simulink model "BatteryStoragePVPlantGFM"  (R2023a)
settings: Solver=FixedStepDiscrete  StartTime=0.0  StopTime=SimulationTime  RelTol=1e-3
PreLoadFcn:
  | run('BatteryStoragePVPlantGFMParameters')
undefined symbols (not defined in the file): Array, Base, battery, BatteryInverter, DiscIntNeverNeededParam, ee, Feeder, fRT, GFLBatteryController, GFMBatteryController, Grid, GridTransformer, Line, Load, Load2CB_final, Load2CB_initial, LVRT, maxSoC, maxVdc, minIrrad, minSoC, minVdc, Mpp, olTime, Panel, PVController, PVInverter, PVTransformer, Scenario, SM, SubTransmissionLine, Ts, VSMbase
libraries: ee_lib x51, nesl_utility x45, fl_lib x26, eeGeneralControl x18, simulink x12, eeTransforms x11, slpidlib x8, eePowerMeasurement x5, batteryecm_lib x2, eeTotalHarmonicDistorsion x2, spsLeadLagFilterLib x1, eeSmAC1C x1
(part 1 of 5)
Description:
  | Copyright 2022 - 2023 The MathWorks, Inc.
settings Model: SimulationMode=accelerator  Creator=rajarshd  LastModifiedBy=rajarshd
settings DataIOCC: InitialState=op  SaveOutput=off  SaveTime=off  ReturnWorkspaceOutputs=off  SignalLoggingName=logs_ee_spv_park_battery
settings OptimizationCC: ReuseModelBlockBuffer=off
settings ModelReferenceCC: EnableRefExpFcnMdlSchedulingChecks=on
settings SimscapeCC: SimscapeLogType=all  SimscapeLogSimulationStatistics=on  SimscapeLogName=simlog_ee_spv_park_battery  SimscapeLogLimitData=off  SimscapeOperatingPoint=op

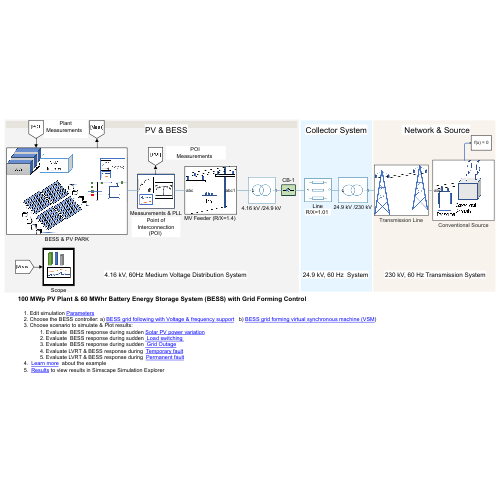
[thumbnail: Simulink's stored preview of the top-level diagram]
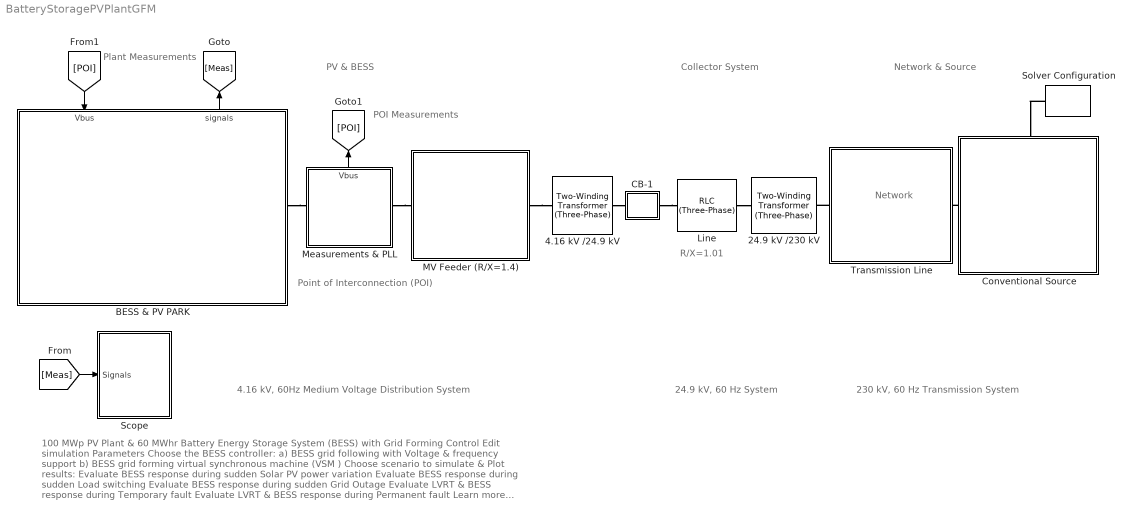
== system BatteryStoragePVPlantGFM ==
  note: Collector System
  note: PV & BESS
  note: Network & Source
  note: Network
  note: 100 MWp PV Plant & 60 MWhr Battery Energy Storage System (BESS) with Grid Forming Control
      |
      | Edit simulation Parameters
      | Choose the BESS controller: a) BESS grid following with Voltage & frequency support b) BESS grid forming virtual synchronous machine (VSM )
      | Choose scenario to simulate & Plot results:
      | Evaluate BESS response during sudden Solar PV power variation
      | Evaluate BESS response during sudden Load switching
      | Evaluate BESS response during sudden Grid Outage
      | Evaluate LVRT & BESS response during Temporary fault
      | Evaluate LVRT & BESS response during Permanent fault
      | Learn more about the example
      | Results to view results in Simscape Simulation Explorer
  note: Point of Interconnection (POI)
  note: 230 kV, 60 Hz Transmission System
  note: 4.16 kV, 60Hz Medium Voltage Distribution System
  note: 24.9 kV, 60 Hz System
  note: R/X=1.01
  note: Plant
      | Measurements
  note: POI
      | Measurements
  24.9 kV /230 kV : ee_lib/Passive/Transformers/Two-Winding Transformer (Three-Phase)  SRated=GridTransformer.VA A*V  FRated=Grid.frequency Hz  Winding1Connection=ee.enum.windingconnection.delta1  VRated1=GridTransformer.hv V  Winding2Connection=ee.enum.windingconnection.Yg  VRated2=GridTransformer.lv V  CoreType=ee.enum.coretype.threelimb  pu_Rw1=GridTransformer.winding_resistance/2  pu_Rw2=GridTransformer.winding_resistance/2  leakage_reactance_option=ee.enum.transformer_leakage.include  pu_Xl1=GridTransformer.winding_lekage_reactance/2  pu_Xl2=GridTransformer.winding_lekage_reactance/2  magnetizing_resistance_option=ee.enum.transformer_magnetizingResistance.exclude  pu_Rm=500  magnetizing_reactance_option=ee.enum.transformer_magnetizingReactance.exclude  saturation_option=ee.enum.transformer_saturation.exclude  pu_Xm=500  current_data=[0, .002, 1, 2]  magnetic_flux_data=[0, 1.2, 1.5, 1.51]  pu_X0=GridTransformer.zero_sequence_reactance  i1_specify=off  i1_priority=None  i1=[0, 0, 0] A  i1_nominal_specify=off  i1_nominal_unit=A  i1_nominal_value=1  i2_specify=off  i2_priority=None  i2=[0, 0, 0] A  i2_nominal_specify=off  i2_nominal_unit=A  i2_nominal_value=1  phi_specify=off  phi_priority=None  phi=[0, 0, 0]  phi_nominal_specify=off  phi_nominal_unit=1  phi_nominal_value=1  power_dissipated_specify=off  power_dissipated_priority=None  power_dissipated=0 W  power_dissipated_nominal_specify=off  power_dissipated_nominal_unit=W  power_dissipated_nominal_value=1
      settings: InternalSimscapePortConfiguration="{\"Bottom\":[],\"Left\":[{\"id\":\"N1\",\"label\":\"~1\",\"type\":\"foundation.electrical.three_phase\"}],\"Right\":[{\"id\":\"N2\",\"label\":\"~2\",\"type\":\"foundation.electrical.three_phase\"}],\"Top\":[]}"
  4.16 kV /24.9 kV : ee_lib/Passive/Transformers/Two-Winding Transformer (Three-Phase)  SRated=PVTransformer.VA A*V  FRated=Grid.frequency Hz  Winding1Connection=ee.enum.windingconnection.delta1  VRated1=PVTransformer.hv V  Winding2Connection=ee.enum.windingconnection.Yg  VRated2=PVTransformer.lv V  CoreType=ee.enum.coretype.threelimb  pu_Rw1=PVTransformer.winding_resistance/2  pu_Rw2=PVTransformer.winding_resistance/2  leakage_reactance_option=ee.enum.transformer_leakage.include  pu_Xl1=PVTransformer.winding_lekage_reactance/2  pu_Xl2=PVTransformer.winding_lekage_reactance/2  magnetizing_resistance_option=ee.enum.transformer_magnetizingResistance.exclude  pu_Rm=500  magnetizing_reactance_option=ee.enum.transformer_magnetizingReactance.exclude  saturation_option=ee.enum.transformer_saturation.exclude  pu_Xm=500  current_data=[0, .002, 1, 2]  magnetic_flux_data=[0, 1.2, 1.5, 1.51]  pu_X0=PVTransformer.zero_sequence_reactance  i1_specify=off  i1_priority=None  i1=[0, 0, 0] A  i1_nominal_specify=off  i1_nominal_unit=A  i1_nominal_value=1  i2_specify=off  i2_priority=None  i2=[0, 0, 0] A  i2_nominal_specify=off  i2_nominal_unit=A  i2_nominal_value=1  phi_specify=off  phi_priority=None  phi=[0, 0, 0]  phi_nominal_specify=off  phi_nominal_unit=1  phi_nominal_value=1  power_dissipated_specify=off  power_dissipated_priority=None  power_dissipated=0 W  power_dissipated_nominal_specify=off  power_dissipated_nominal_unit=W  power_dissipated_nominal_value=1
      settings: InternalSimscapePortConfiguration="{\"Bottom\":[],\"Left\":[{\"id\":\"N1\",\"label\":\"~1\",\"type\":\"foundation.electrical.three_phase\"}],\"Right\":[{\"id\":\"N2\",\"label\":\"~2\",\"type\":\"foundation.electrical.three_phase\"}],\"Top\":[]}"
  BESS & PV PARK : Subsystem
      settings: PortSchema="{\"entries\":[{\"content\":{\"sides\":[{\"content\":{\"connectorIds\":[]},\"type\":\"ConnectorPlacement.EquallySpacedRectSide\",\"uuid\":\"19e6e0fd-37ae-4388-8e0e-5a20feba0fd4\"},{\"content\":{\"connectorIds\":[\"RConn1\"],\"side\":\"RIGHT\"},\"type\":\"ConnectorPlacement.EquallySpacedRectSide\",\"uuid\":\"5a7c928c-05b2-4ad3-8813-df6fbac671b7\"},{\"content\":{\"connectorIds\":[\"In1\",\"Out1\"],\"side\":\"TOP\"},\"type\":\"ConnectorPlacement.EquallySpacedRectSide\",\"uuid\":\"fc17c31c-808c-4646-acd6-16363c98e490\"}]},\"type\":\"ConnectorPlacement.EquallySpacedConnector\",\"uuid\":\"d03db955-298f-40d1-b8c3-c83724e206fe\"}],\"packageUris\":[\"http://schema.mathworks.com/mf0/Connector/R2020b\"],\"version\":\"1.0\"}"
      mask Display: image('$imagefile'); % Use "Edit Image" on toolstrip to change.
  CB-1 : Subsystem
      mask Display: image('$imagefile'); % Use "Edit Image" on toolstrip to change.
  Conventional Source : Subsystem
      settings: PortSchema="{\"entries\":[{\"content\":{\"sides\":[{\"content\":{\"connectorIds\":[\"LConn1\"]},\"type\":\"ConnectorPlacement.EquallySpacedRectSide\",\"uuid\":\"88e24179-6079-4110-b6c8-07285d357c8a\"},{\"content\":{\"connectorIds\":[],\"side\":\"RIGHT\"},\"type\":\"ConnectorPlacement.EquallySpacedRectSide\",\"uuid\":\"8f4b6582-111e-4598-90a5-fa5f81c444ee\"},{\"content\":{\"connectorIds\":[\"LConn2\"],\"side\":\"TOP\"},\"type\":\"ConnectorPlacement.EquallySpacedRectSide\",\"uuid\":\"53212e71-0f3c-4549-bc92-047e88eae9b6\"},{\"content\":{\"connectorIds\":[],\"side\":\"BOTTOM\"},\"type\":\"ConnectorPlacement.EquallySpacedRectSide\",\"uuid\":\"0193069a-d0a5-4b89-8f2a-3f6fb986b7f7\"}]},\"type\":\"ConnectorPlacement.EquallySpacedConnector\",\"uuid\":\"b2543555-7807-483c-9e73-a2cd2a98a3a5\"}],\"packageUris\":[\"http://schema.mathworks.com/mf0/Connector/R2020b\"],\"version\":\"1.0\"}"
      mask Display: image('$imagefile'); % Use "Edit Image" on toolstrip to change.
  Line : ee_lib/Passive/RLC Assemblies/RLC (Three-Phase)  component_structure=ee.enum.rlc.structure.SeriesRL  R=SubTransmissionLine.R*SubTransmissionLine.length Ohm  L=SubTransmissionLine.L*SubTransmissionLine.length H  C=1e-6 F  R_parasitic=0 Ohm  G_parasitic=0 1/Ohm  IL_specify=off  IL_priority=High  IL=[0, 0, 0] A  IL_nominal_specify=off  IL_nominal_unit=A  IL_nominal_value=1  VC_specify=off  VC_priority=High  VC=[0, 0, 0] V  VC_nominal_specify=off  VC_nominal_unit=V  VC_nominal_value=1
      settings: InternalSimscapePortConfiguration="{\"Bottom\":[],\"Left\":[{\"id\":\"N1\",\"label\":\"~1\",\"type\":\"foundation.electrical.three_phase\"}],\"Right\":[{\"id\":\"N2\",\"label\":\"~2\",\"type\":\"foundation.electrical.three_phase\"}],\"Top\":[]}"
  "MV Feeder (R/X=1.4) " : Subsystem
      mask Display: image('$imagefile'); % Use "Edit Image" on toolstrip to change.
  Measurements & PLL : Subsystem
      settings: PortSchema="{\"entries\":[{\"content\":{\"sides\":[{\"content\":{\"connectorIds\":[\"LConn1\"]},\"type\":\"ConnectorPlacement.EquallySpacedRectSide\",\"uuid\":\"0a665b18-901e-42b1-b0d0-6060e0da8e79\"},{\"content\":{\"connectorIds\":[\"RConn1\"],\"side\":\"RIGHT\"},\"type\":\"ConnectorPlacement.EquallySpacedRectSide\",\"uuid\":\"7ff1075b-9d20-42a5-b79b-99217310976a\"},{\"content\":{\"connectorIds\":[\"Out1\"],\"side\":\"TOP\"},\"type\":\"ConnectorPlacement.EquallySpacedRectSide\",\"uuid\":\"7168f638-c3c0-42b4-ab34-d46b363fbd60\"},{\"content\":{\"connectorIds\":[],\"side\":\"BOTTOM\"},\"type\":\"ConnectorPlacement.EquallySpacedRectSide\",\"uuid\":\"9ec0f51f-0ad1-4b03-97b0-093edc8b098b\"}]},\"type\":\"ConnectorPlacement.EquallySpacedConnector\",\"uuid\":\"d15f0547-e531-4cb7-ae74-94ae676078ed\"}],\"packageUris\":[\"http://schema.mathworks.com/mf0/Connector/R2020b\"],\"version\":\"1.0\"}"
      mask Display: image('$imagefile'); % Use "Edit Image" on toolstrip to change.
  Scope : Subsystem
      mask Display: image('$imagefile'); % Use "Edit Image" on toolstrip to change.
  Solver Configuration : nesl_utility/Solver Configuration  PhysicalDomain=network_engine_domain  SubClassName=solver  LeftPortType=input  RightPortType=generic  Tones=[]  Harmonics=[]  SimulateNoise=off  Profile=off  UseLocalSampling=off  EnableSwitchedLinearOptims=on  FrequencyDomain=off  UseCCode=off  RelTol=0.001  AbsTol=1e-06  MinStep=1e-09  ToWorkspace=off  RevertToSquareIcSolve=off  NumHomotopyIterations=100  PhasorMode=off  PhasorModeNumHarmonics=1  ConsistencySolver=NEWTON_FTOL  IndexReductionMethod=DerivativeReplacement  DoDC=off  ResidualTolerance=1e-09  ConsistencyTolSource=GLOBAL  ConsistencyAbsTol=0.001  ConsistencyRelTol=0.001  ConsistencyTolFactor=0.001  UseLocalSolver=on  LocalSolverChoice=NE_PARTITIONING_ADVANCER  ResolveIndetEquations=on  FunctionEvalNumThread=1  LocalSolverSampleTime=Ts  DoFixedCost=on  MaxNonlinIter=3  MaxModeIter=2  ComputeImpulses=off  ImpulseIterations=2  LinearAlgebra=auto  LinearAlgebraNumThread=0  EquationFormulation=NE_TIME_EF  DelaysMemoryBudget=1024  AutomaticFiltering=on  FilteringTimeConstant=0.001  PartitionStorageMethod=AS_NEEDED  PartitionMemoryBudget=1024  PartitionMethod=ROBUST
  Transmission Line : Subsystem
      mask Display: image('$imagefile'); % Use "Edit Image" on toolstrip to change.
  wires:
  [Meas] -> Scope/1(Signals)
  Measurements & PLL/1(Vbus) -> [POI]
  [POI] -> BESS & PV PARK/1(Vbus)
  BESS & PV PARK/1(signals) -> [Meas]
  connections:
  Transmission Line/LConn1 -- 24.9 kV /230 kV/LConn1
  BESS & PV PARK/RConn1 -- Measurements & PLL/LConn1
  Measurements & PLL/RConn1 -- "MV Feeder (R/X=1.4) "/LConn1
  "MV Feeder (R/X=1.4) "/RConn1 -- 4.16 kV /24.9 kV/RConn1
  Conventional Source/LConn1 -- Transmission Line/RConn1
  Solver Configuration/RConn1 -- Conventional Source/LConn2
  4.16 kV /24.9 kV/LConn1 -- CB-1/LConn1
  CB-1/RConn1 -- Line/LConn1
  Line/RConn1 -- 24.9 kV /230 kV/RConn1

== system BatteryStoragePVPlantGFM/BESS & PV PARK ==
  note: Voltage & Current
      | Measurements
  note: Voltage & Current
      | Measurements
  In Bus Element : Inport  PortName=Vbus
  100 MWp PV Park : Subsystem
      settings: PortSchema="{\"entries\":[{\"content\":{\"sides\":[{\"content\":{\"connectorIds\":[\"Out1\",\"In1\",\"LConn1\"]},\"type\":\"ConnectorPlacement.EquallySpacedRectSide\",\"uuid\":\"343ce997-9cac-43fa-9216-298045fd67dd\"},{\"content\":{\"connectorIds\":[\"In2\",\"In3\"],\"side\":\"RIGHT\"},\"type\":\"ConnectorPlacement.EquallySpacedRectSide\",\"uuid\":\"419648e9-cc51-43b2-af12-d3f937f2b6d1\"},{\"content\":{\"connectorIds\":[],\"side\":\"TOP\"},\"type\":\"ConnectorPlacement.EquallySpacedRectSide\",\"uuid\":\"296a2476-614b-49ee-a38a-605419a1856a\"},{\"content\":{\"connectorIds\":[],\"side\":\"BOTTOM\"},\"type\":\"ConnectorPlacement.EquallySpacedRectSide\",\"uuid\":\"1a94dbbe-b4b3-4e2f-8128-897afc680bd0\"}]},\"type\":\"ConnectorPlacement.EquallySpacedConnector\",\"uuid\":\"83a42d0e-456a-4e37-b942-9ac5d756f0ba\"}],\"packageUris\":[\"http://schema.mathworks.com/mf0/Connector/R2020b\"],\"version\":\"1.0\"}"
      mask Display: image('$imagefile'); % Use "Edit Image" on toolstrip to change.
  60 MWhr Battery Energy Storage : Subsystem
      settings: PortSchema="{\"entries\":[{\"content\":{\"sides\":[{\"content\":{\"connectorIds\":[\"In1\"]},\"type\":\"ConnectorPlacement.EquallySpacedRectSide\",\"uuid\":\"883e7b19-0e26-46af-952e-c8bc8ad7c7c8\"},{\"content\":{\"connectorIds\":[\"RConn1\",\"In2\",\"Out1\"],\"side\":\"RIGHT\"},\"type\":\"ConnectorPlacement.EquallySpacedRectSide\",\"uuid\":\"7a83414d-eb58-4460-b24e-307c8bde3358\"},{\"content\":{\"connectorIds\":[],\"side\":\"TOP\"},\"type\":\"ConnectorPlacement.EquallySpacedRectSide\",\"uuid\":\"c6d607b7-7e86-4905-bc25-9c78b4ff15f7\"},{\"content\":{\"connectorIds\":[],\"side\":\"BOTTOM\"},\"type\":\"ConnectorPlacement.EquallySpacedRectSide\",\"uuid\":\"e1bc4c26-6ec5-4df0-8f96-867ea0072814\"}]},\"type\":\"ConnectorPlacement.EquallySpacedConnector\",\"uuid\":\"ef2fc235-7b9f-436b-9d0c-7c76d6f36368\"}],\"packageUris\":[\"http://schema.mathworks.com/mf0/Connector/R2020b\"],\"version\":\"1.0\"}"
      mask Display: image('$imagefile'); % Use "Edit Image" on toolstrip to change.
  CB-3 : Subsystem
      settings: PortSchema="{\"entries\":[{\"content\":{\"sides\":[{\"content\":{\"connectorIds\":[\"LConn1\"]},\"type\":\"ConnectorPlacement.EquallySpacedRectSide\",\"uuid\":\"89547ea5-ae6b-4d0f-97d1-dbb6906b1f5d\"},{\"content\":{\"connectorIds\":[\"RConn1\"],\"side\":\"RIGHT\"},\"type\":\"ConnectorPlacement.EquallySpacedRectSide\",\"uuid\":\"0d1aef66-c8e0-4a24-b797-81618e5184b2\"},{\"content\":{\"connectorIds\":[],\"side\":\"TOP\"},\"type\":\"ConnectorPlacement.EquallySpacedRectSide\",\"uuid\":\"90b9d15b-1652-4bf4-b42a-4b1767bf3ee6\"},{\"content\":{\"connectorIds\":[\"In1\"],\"side\":\"BOTTOM\"},\"type\":\"ConnectorPlacement.EquallySpacedRectSide\",\"uuid\":\"eff9f7f6-ab14-4529-b757-a609d833a6df\"}]},\"type\":\"ConnectorPlacement.EquallySpacedConnector\",\"uuid\":\"9555d053-edbd-4f07-b819-a60b35f35e2e\"}],\"packageUris\":[\"http://schema.mathworks.com/mf0/Connector/R2020b\"],\"version\":\"1.0\"}"
      mask Display: image('$imagefile'); % Use "Edit Image" on toolstrip to change.
  CB-4 : Subsystem
      settings: PortSchema="{\"entries\":[{\"content\":{\"sides\":[{\"content\":{\"connectorIds\":[\"LConn1\"]},\"type\":\"ConnectorPlacement.EquallySpacedRectSide\",\"uuid\":\"89547ea5-ae6b-4d0f-97d1-dbb6906b1f5d\"},{\"content\":{\"connectorIds\":[\"RConn1\"],\"side\":\"RIGHT\"},\"type\":\"ConnectorPlacement.EquallySpacedRectSide\",\"uuid\":\"0d1aef66-c8e0-4a24-b797-81618e5184b2\"},{\"content\":{\"connectorIds\":[\"In1\"],\"side\":\"TOP\"},\"type\":\"ConnectorPlacement.EquallySpacedRectSide\",\"uuid\":\"90b9d15b-1652-4bf4-b42a-4b1767bf3ee6\"}]},\"type\":\"ConnectorPlacement.EquallySpacedConnector\",\"uuid\":\"9555d053-edbd-4f07-b819-a60b35f35e2e\"}],\"packageUris\":[\"http://schema.mathworks.com/mf0/Connector/R2020b\"],\"version\":\"1.0\"}"
      mask Display: image('$imagefile'); % Use "Edit Image" on toolstrip to change.
  "PV Plant Controller " : Subsystem
      settings: PortSchema="{\"entries\":[{\"content\":{\"sides\":[{\"content\":{\"connectorIds\":[\"In1\"]},\"type\":\"ConnectorPlacement.EquallySpacedRectSide\",\"uuid\":\"4dd5c331-822d-4333-9dd3-7a69fe680142\"},{\"content\":{\"connectorIds\":[\"In2\",\"Out1\",\"Out2\",\"Out3\",\"Out4\",\"In3\"],\"side\":\"RIGHT\"},\"type\":\"ConnectorPlacement.EquallySpacedRectSide\",\"uuid\":\"85556e6f-552b-436d-96c5-f50473e6eef2\"},{\"content\":{\"connectorIds\":[],\"side\":\"TOP\"},\"type\":\"ConnectorPlacement.EquallySpacedRectSide\",\"uuid\":\"5ac869aa-0c48-488d-8d32-cb0a103032a5\"}]},\"type\":\"ConnectorPlacement.EquallySpacedConnector\",\"uuid\":\"1c77cf04-edee-41fe-a91f-465f3e8ec46b\"}],\"packageUris\":[\"http://schema.mathworks.com/mf0/Connector/R2020b\"],\"version\":\"1.0\"}"
      mask Display: image('$imagefile'); % Use "Edit Image" on toolstrip to change.
  Conn1 : PMIOPort  Side=Right
  signals : Outport
  wires:
  In Bus Element/1 -> "PV Plant Controller "/1(Vbus), 100 MWp PV Park/2(Vbus), 60 MWhr Battery Energy Storage/1(Vbus)
  [trip] -> CB-3/1(Input)
  100 MWp PV Park/1(IPV) -> "PV Plant Controller "/3(IPV)
  [LVRT_iq] -> 60 MWhr Battery Energy Storage/2(Input)
  [LVRT_iq] -> 100 MWp PV Park/1(LVRT_iq)
  "PV Plant Controller "/2(LVRT.breaker) -> [trip]
  "PV Plant Controller "/1(LVRT_iq) -> [LVRT_iq]
  60 MWhr Battery Energy Storage/1(Bat) -> "PV Plant Controller "/2(Bat)
  [trip] -> CB-4/1(Input)
  "PV Plant Controller "/3(signals) -> signals/1
  "PV Plant Controller "/4(Q_ref) -> [Q_ref]
  [Q_ref] -> 100 MWp PV Park/3(Q_ref)
  connections:
  100 MWp PV Park/LConn1 -- CB-4/LConn1
  CB-3/RConn1 -- Conn1/RConn1 -- CB-4/RConn1
  CB-3/LConn1 -- 60 MWhr Battery Energy Storage/RConn1

== system BatteryStoragePVPlantGFM/CB-1 ==
  Circuit Breaker Step off3 : ee_lib/Switches & Breakers/Circuit Breaker (Three-Phase)  R_closed=0.001 Ohm  G_open=1e-4 1/Ohm  threshold=0.5 V  breaker_behavior=ee.enum.switches.breakerBehavior.zeroCrossingEnable
      settings: InternalSimscapePortConfiguration="{\"Bottom\":[],\"Left\":[{\"id\":\"vT\",\"label\":\"vT\",\"type\":\"input\"},{\"id\":\"N1\",\"label\":\"~1\",\"type\":\"foundation.electrical.three_phase\"}],\"Right\":[{\"id\":\"N2\",\"label\":\"~2\",\"type\":\"foundation.electrical.three_phase\"}],\"Top\":[]}"
  Simulink-PS Converter3 : nesl_utility/Simulink-PS Converter  PhysicalDomain=network_engine_domain  SubClassName=ps_input  LeftPortType=input  RightPortType=output  PseudoPeriodic=off  Frequencies=[]  NoiseDistribution=none  NoiseParameters=[]  Unit=1  AffineConversion=off  FilteringAndDerivatives=zero  SimscapeFilterOrder=1  InputFilterTimeConstant=0.001  UdotUserProvided=1
  Step off3 : Step  Time=Scenario.Grid_outage_time  SampleTime=Ts
  Conn2 : PMIOPort  Side=Left
  Conn1 : PMIOPort  Port=2  Side=Right
  wires:
  Step off3/1 -> Simulink-PS Converter3/1
  connections:
  Circuit Breaker Step off3/LConn2 -- Conn2/RConn1
  Circuit Breaker Step off3/LConn1 -- Simulink-PS Converter3/RConn1
  Circuit Breaker Step off3/RConn1 -- Conn1/RConn1

== system BatteryStoragePVPlantGFM/Conventional Source ==
  Current and Voltage Sensor (Three-Phase)4 : ee_lib/Sensors & Transducers/Current and Voltage Sensor (Three-Phase)  vMeasurementType=ee.enum.vmeasurement.lg  outputUnit=ee.enum.unit.si  SRated=Base.MVA_base_new A*V  VRated=Base.KV_base_new V  I_specify=off  I_priority=None  I=[0, 0, 0] A  I_nominal_specify=off  I_nominal_unit=A  I_nominal_value=1  V_specify=off  V_priority=None  V=[0, 0, 0] V  V_nominal_specify=off  V_nominal_unit=V  V_nominal_value=1
      settings: InternalSimscapePortConfiguration="{\"Bottom\":[],\"Left\":[{\"id\":\"N1\",\"label\":\"~1\",\"type\":\"foundation.electrical.three_phase\"}],\"Right\":[{\"id\":\"V_output\",\"label\":\"V\",\"type\":\"output\"},{\"id\":\"I_output\",\"label\":\"I\",\"type\":\"output\"},{\"id\":\"N2\",\"label\":\"~2\",\"type\":\"foundation.electrical.three_phase\"}],\"Top\":[]}"
  Measurements : Subsystem
  PS-Simulink Converter2 : nesl_utility/PS-Simulink Converter  PhysicalDomain=network_engine_domain  SubClassName=ps_output  LeftPortType=input  RightPortType=output  PseudoPeriodic=off  Frequencies=[]  VectorFormat=inherit  Unit=inherit  AffineConversion=off
  PS-Simulink Converter3 : nesl_utility/PS-Simulink Converter  PhysicalDomain=network_engine_domain  SubClassName=ps_output  LeftPortType=input  RightPortType=output  PseudoPeriodic=off  Frequencies=[]  VectorFormat=inherit  Unit=inherit  AffineConversion=off
  Variant Subsystem : Subsystem  Variant=on
  abc : PMIOPort  Side=Left
  Connection Port : PMIOPort  Port=2  Side=Left
  wires:
  PS-Simulink Converter3/1 -> Measurements/2(I)
  Measurements/1(Grid) -> Variant Subsystem/1(Grid)
  PS-Simulink Converter2/1 -> Measurements/1(V)
  connections:
  Current and Voltage Sensor (Three-Phase)4/RConn3 -- abc/RConn1
  PS-Simulink Converter2/LConn1 -- Current and Voltage Sensor (Three-Phase)4/RConn1
  PS-Simulink Converter3/LConn1 -- Current and Voltage Sensor (Three-Phase)4/RConn2
  Variant Subsystem/RConn1 -- Current and Voltage Sensor (Three-Phase)4/LConn1
  Connection Port/RConn1 -- Variant Subsystem/LConn1

== system BatteryStoragePVPlantGFM/MV Feeder (R//X=1.4)  ==
  " Load" : ee_lib/Passive/RLC Assemblies/Wye-Connected Load  parameterization=ee.enum.rlc.parameterization.ratedpower  component_structure=ee.enum.rlc.structure.R  component_structure_PQ=ee.enum.rlc.structure.ParallelRL  R=1 Ohm  L=1e-3 H  C=1e-6 F  VRated=PVTransformer.lv V  FRated=Grid.frequency Hz  P=Load.P1 W  Qpos=Load.Q1 A*V  Qneg=-1e2 A*V  R_parasitic=0 Ohm  G_parasitic=0 1/Ohm  R_parasitic_PQ=0 Ohm  G_parasitic_PQ=0 1/Ohm  Vmag0=4.16e3 V  Vang0=0 deg  Freq0=60 Hz  IL_specify=off  IL_priority=High  IL=[0, 0, 0] A  IL_nominal_specify=off  IL_nominal_unit=A  IL_nominal_value=1  VC_specify=off  VC_priority=High  VC=[0, 0, 0] V  VC_nominal_specify=off  VC_nominal_unit=V  VC_nominal_value=1
  CB1 : Subsystem
      mask Display: image('$imagefile'); % Use "Edit Image" on toolstrip to change.
  CB10 : Subsystem
      mask Display: image('$imagefile'); % Use "Edit Image" on toolstrip to change.
  Electrical Reference1 : fl_lib/Electrical/Electrical Elements/Electrical Reference
  Electrical Reference2 : fl_lib/Electrical/Electrical Elements/Electrical Reference
  Feeder (R/X=1.4)1 : ee_lib/Passive/RLC Assemblies/RLC (Three-Phase)  component_structure=ee.enum.rlc.structure.SeriesRL  R=(Feeder.R_f)*Feeder.lengthSecondHalf Ohm  L=(Feeder.L_f)*Feeder.lengthSecondHalf H  C=1e-6 F  R_parasitic=0 Ohm  G_parasitic=0 1/Ohm  IL_specify=off  IL_priority=High  IL=[0, 0, 0] A  IL_nominal_specify=off  IL_nominal_unit=A  IL_nominal_value=1  VC_specify=off  VC_priority=High  VC=[0, 0, 0] V  VC_nominal_specify=off  VC_nominal_unit=V  VC_nominal_value=1
      settings: InternalSimscapePortConfiguration="{\"Bottom\":[],\"Left\":[{\"id\":\"N1\",\"label\":\"~1\",\"type\":\"foundation.electrical.three_phase\"}],\"Right\":[{\"id\":\"N2\",\"label\":\"~2\",\"type\":\"foundation.electrical.three_phase\"}],\"Top\":[]}"
  Feeder (R/X=1.4)2 : ee_lib/Passive/RLC Assemblies/RLC (Three-Phase)  component_structure=ee.enum.rlc.structure.SeriesRL  R=Feeder.R_f*Feeder.lengthFirstHalf Ohm  L=Feeder.L_f*Feeder.lengthFirstHalf H  C=1e-6 F  R_parasitic=0 Ohm  G_parasitic=0 1/Ohm  IL_specify=off  IL_priority=High  IL=[0, 0, 0] A  IL_nominal_specify=off  IL_nominal_unit=A  IL_nominal_value=1  VC_specify=off  VC_priority=High  VC=[0, 0, 0] V  VC_nominal_specify=off  VC_nominal_unit=V  VC_nominal_value=1
      settings: InternalSimscapePortConfiguration="{\"Bottom\":[],\"Left\":[{\"id\":\"N1\",\"label\":\"~1\",\"type\":\"foundation.electrical.three_phase\"}],\"Right\":[{\"id\":\"N2\",\"label\":\"~2\",\"type\":\"foundation.electrical.three_phase\"}],\"Top\":[]}"
  Load1 : ee_lib/Passive/RLC Assemblies/Wye-Connected Load  parameterization=ee.enum.rlc.parameterization.ratedpower  component_structure=ee.enum.rlc.structure.R  component_structure_PQ=ee.enum.rlc.structure.ParallelRL  R=1 Ohm  L=1e-3 H  C=1e-6 F  VRated=PVTransformer.lv V  FRated=Grid.frequency Hz  P=Load.P2 W  Qpos=Load.Q2 A*V  Qneg=-1e2 A*V  R_parasitic=0 Ohm  G_parasitic=0 1/Ohm  R_parasitic_PQ=0 Ohm  G_parasitic_PQ=0 1/Ohm  Vmag0=4.16e3 V  Vang0=0 deg  Freq0=60 Hz  IL_specify=off  IL_priority=High  IL=[0, 0, 0] A  IL_nominal_specify=off  IL_nominal_unit=A  IL_nominal_value=1  VC_specify=off  VC_priority=High  VC=[0, 0, 0] V  VC_nominal_specify=off  VC_nominal_unit=V  VC_nominal_value=1
  abc : PMIOPort  Side=Left
  abc1 : PMIOPort  Port=2  Side=Right
  connections:
  " Load"/LConn1 -- CB10/RConn1
  Feeder (R/X=1.4)1/RConn1 -- abc1/RConn1
  CB10/LConn1 -- Feeder (R/X=1.4)1/LConn1 -- CB1/LConn1 -- Feeder (R/X=1.4)2/RConn1
  Feeder (R/X=1.4)2/LConn1 -- abc/RConn1
  Electrical Reference1/LConn1 -- " Load"/RConn1
  Electrical Reference2/LConn1 -- Load1/RConn1
  Load1/LConn1 -- CB1/RConn1

== system BatteryStoragePVPlantGFM/Measurements & PLL ==
  Current and Voltage Sensor (Three-Phase)5 : ee_lib/Sensors & Transducers/Current and Voltage Sensor (Three-Phase)  vMeasurementType=ee.enum.vmeasurement.lg  outputUnit=ee.enum.unit.pu  SRated=Base.MVA_base_new A*V  VRated=Base.KV_base_new V  I_specify=off  I_priority=None  I=[0, 0, 0] A  I_nominal_specify=off  I_nominal_unit=A  I_nominal_value=1  V_specify=off  V_priority=None  V=[0, 0, 0] V  V_nominal_specify=off  V_nominal_unit=V  V_nominal_value=1
      settings: InternalSimscapePortConfiguration="{\"Bottom\":[],\"Left\":[{\"id\":\"N1\",\"label\":\"~1\",\"type\":\"foundation.electrical.three_phase\"}],\"Right\":[{\"id\":\"V_output\",\"label\":\"V\",\"type\":\"output\"},{\"id\":\"I_output\",\"label\":\"I\",\"type\":\"output\"},{\"id\":\"N2\",\"label\":\"~2\",\"type\":\"foundation.electrical.three_phase\"}],\"Top\":[]}"
  Demux : Demux  Outputs=3
  Demux1 : Demux  Outputs=3
  Display : Display
  Display1 : Display
  PLL & Measurements : Subsystem
      settings: PortSchema="{\"entries\":[{\"content\":{\"sides\":[{\"content\":{\"connectorIds\":[\"Out1\",\"In1\",\"In2\"]},\"type\":\"ConnectorPlacement.EquallySpacedRectSide\",\"uuid\":\"76485780-20fe-4fcf-8224-69648da6ed2a\"},{\"content\":{\"connectorIds\":[],\"side\":\"RIGHT\"},\"type\":\"ConnectorPlacement.EquallySpacedRectSide\",\"uuid\":\"f19a6390-e634-42c7-8d46-4cd80cbab182\"},{\"content\":{\"connectorIds\":[],\"side\":\"TOP\"},\"type\":\"ConnectorPlacement.EquallySpacedRectSide\",\"uuid\":\"87682f72-1844-428e-be70-ad7ca3191ee3\"}]},\"type\":\"ConnectorPlacement.EquallySpacedConnector\",\"uuid\":\"f2136b07-48ec-402b-adb3-18c0bac2157c\"}],\"packageUris\":[\"http://schema.mathworks.com/mf0/Connector/R2020b\"],\"version\":\"1.0\"}"
      mask Display: image('$imagefile'); % Use "Edit Image" on toolstrip to change.
  PS-Simulink Converter1 : nesl_utility/PS-Simulink Converter  PhysicalDomain=network_engine_domain  SubClassName=ps_output  LeftPortType=input  RightPortType=output  PseudoPeriodic=off  Frequencies=[]  VectorFormat=inherit  Unit=inherit  AffineConversion=off
  PS-Simulink Converter2 : nesl_utility/PS-Simulink Converter  PhysicalDomain=network_engine_domain  SubClassName=ps_output  LeftPortType=input  RightPortType=output  PseudoPeriodic=off  Frequencies=[]  VectorFormat=inherit  Unit=inherit  AffineConversion=off
  Terminator{,1..3} (4 alike) : Terminator
  Total Harmonic Distortion : eeTotalHarmonicDistorsion/Total Harmonic Distortion  f=Grid.frequency  Ts=Ts
      settings: LibrarySourceBlock=|
      | ee_sl_lib/Measurements/Total Harmonic
      | Distortion
  Total Harmonic Distortion1 : eeTotalHarmonicDistorsion/Total Harmonic Distortion  f=Grid.frequency  Ts=Ts
      settings: LibrarySourceBlock=|
      | ee_sl_lib/Measurements/Total Harmonic
      | Distortion
  abc : PMIOPort  Side=Left
  abc1 : PMIOPort  Port=2  Side=Right
  Vbus : Outport
  wires:
  PLL & Measurements/1(Vbus) -> Vbus/1
  PS-Simulink Converter1/1 -> Demux/1, PLL & Measurements/2(I)
  Total Harmonic Distortion/1 -> Display/1
  Total Harmonic Distortion1/1 -> Display1/1
  Demux/1 -> Total Harmonic Distortion/1
  Demux/3 -> Terminator/1
  Demux/2 -> Terminator1/1
  Demux1/1 -> Total Harmonic Distortion1/1
  PS-Simulink Converter2/1 -> Demux1/1, PLL & Measurements/1(V)
  Demux1/2 -> Terminator2/1
  Demux1/3 -> Terminator3/1
  connections:
  abc1/RConn1 -- Current and Voltage Sensor (Three-Phase)5/RConn3
  abc/RConn1 -- Current and Voltage Sensor (Three-Phase)5/LConn1
  PS-Simulink Converter1/LConn1 -- Current and Voltage Sensor (Three-Phase)5/RConn2
  PS-Simulink Converter2/LConn1 -- Current and Voltage Sensor (Three-Phase)5/RConn1

== system BatteryStoragePVPlantGFM/Scope ==
  Signals : Inport
  Bus Selector : BusSelector  OutputSignals=P_total,Q_total,Vmag,w,Vabc,Iabc,P_Bat,Q_Bat,P_PV,Q_PV,Iabc_bat
  Gain{,1..5} (6 alike) : Gain  Gain=10^-6
  Gain6 : Gain  Gain=25/90
  Gain7 : Gain  Gain=(sqrt(3)*Base.KV_base_new)/battery.baseMVA
  Scope : Scope  NumInputPorts=11
  wires:
  Signals/1 -> Bus Selector/1
  Bus Selector/1 -> Gain/1  "<P_total>"
  Bus Selector/2 -> Gain1/1  "<Q_total>"
  Bus Selector/6 -> Gain6/1  "<Iabc>"
  Bus Selector/7 -> Gain5/1  "<P_Bat>"
  Bus Selector/8 -> Gain3/1  "<Q_Bat>"
  Bus Selector/9 -> Gain2/1  "<P_PV>"
  Bus Selector/10 -> Gain4/1  "<Q_PV>"
  Bus Selector/11 -> Gain7/1  "<Iabc_bat>"
  Gain/1 -> Scope/1
  Gain1/1 -> Scope/2
  Bus Selector/3 -> Scope/3  "<Vmag>"
  Bus Selector/4 -> Scope/4  "<w>"
  Bus Selector/5 -> Scope/5  "<Vabc>"
  Gain6/1 -> Scope/6
  Gain5/1 -> Scope/7
  Gain3/1 -> Scope/8
  Gain2/1 -> Scope/9
  Gain4/1 -> Scope/10
  Gain7/1 -> Scope/11

== system BatteryStoragePVPlantGFM/Transmission Line ==
  CB : Subsystem
      mask Display: image('$imagefile'); % Use "Edit Image" on toolstrip to change.
  CB5 : Subsystem
      mask Display: image('$imagefile'); % Use "Edit Image" on toolstrip to change.
  Electrical Reference{1..4} (4 alike) : fl_lib/Electrical/Electrical Elements/Electrical Reference
  "Fault " : ee_lib/Utilities/Fault (Three-Phase)  fault_type_option=10  R_pn_fault=1e-3 Ohm  R_ng_fault=1e-3 Ohm  exposemeasurement=ee.enum.exposemeasurement.hidden  enable_external_fault=ee.enum.external_fault.hidden  fault_threshold=0.5  fault_condition=1  fault_resettable=0  enable_temporal_fault=1  fault_start_time=Scenario.Fault_time s  fault_duration=Scenario.Fault_duration s  G_parasitic=1e-6 1/Ohm
      settings: InternalSimscapePortConfiguration="{\"Bottom\":[],\"Left\":[{\"id\":\"N\",\"label\":\"~\",\"type\":\"foundation.electrical.three_phase\"}],\"Right\":[],\"Top\":[]}"
  "l Km " : ee_lib/Passive/Lines/Transmission Line (Three-Phase)  length=Line.l_km*Scenario.Fault_distance km  freq=Grid.frequency Hz  R=Line.r_l Ohm/km  L=Line.L_l mH/km  M=Line.M_l mH/km  Cl=Line.C_ll uF/km  Cg=Line.C_lg uF/km  Rm=Line.Mr Ohm/km  N=1  R_parasitic=1e-5 Ohm  G_parasitic=1e-4 1/Ohm  enable_fault=ee.enum.enable.no  fault_type_option=ee.enum.fault_type_option.abc  R_pn_fault=1e-2 Ohm  R_ng_fault=1e-2 Ohm  unfaulted_G_parasitic=1e-6 1/Ohm  length_fault=Line.l_km*Scenario.Fault_distance km  N1_fault=1  N2_fault=1  Access_ground=ee.enum.enable.no
      settings: InternalSimscapePortConfiguration="{\"Bottom\":[],\"Left\":[{\"id\":\"N1\",\"label\":\"~1\",\"type\":\"foundation.electrical.three_phase\"},{\"id\":\"g1\",\"label\":\"g1\",\"type\":\"foundation.electrical.electrical\"}],\"Right\":[{\"id\":\"N2\",\"label\":\"~2\",\"type\":\"foundation.electrical.three_phase\"},{\"id\":\"g2\",\"label\":\"g2\",\"type\":\"foundation.electrical.electrical\"}],\"Top\":[]}"
  "l1 Km " : ee_lib/Passive/Lines/Transmission Line (Three-Phase)  length=Line.l_km*(1-Scenario.Fault_distance) km  freq=Grid.frequency Hz  R=Line.r_l Ohm/km  L=Line.L_l mH/km  M=Line.M_l mH/km  Cl=Line.C_ll uF/km  Cg=Line.C_lg uF/km  Rm=Line.Mr Ohm/km  N=1  R_parasitic=1e-5 Ohm  G_parasitic=1e-4 1/Ohm  enable_fault=ee.enum.enable.no  fault_type_option=ee.enum.fault_type_option.abc  R_pn_fault=1e-2 Ohm  R_ng_fault=1e-2 Ohm  unfaulted_G_parasitic=1e-6 1/Ohm  length_fault=Line.l_km*Scenario.Fault_distance km  N1_fault=1  N2_fault=1  Access_ground=ee.enum.enable.no
      settings: InternalSimscapePortConfiguration="{\"Bottom\":[],\"Left\":[{\"id\":\"N1\",\"label\":\"~1\",\"type\":\"foundation.electrical.three_phase\"},{\"id\":\"g1\",\"label\":\"g1\",\"type\":\"foundation.electrical.electrical\"}],\"Right\":[{\"id\":\"N2\",\"label\":\"~2\",\"type\":\"foundation.electrical.three_phase\"},{\"id\":\"g2\",\"label\":\"g2\",\"type\":\"foundation.electrical.electrical\"}],\"Top\":[]}"
  abc1 : PMIOPort  Side=Right
  abc : PMIOPort  Port=2  Side=Left
  connections:
  CB5/RConn1 -- "l Km "/LConn1
  Electrical Reference1/LConn1 -- "l Km "/RConn2
  CB5/LConn1 -- abc/RConn1
  Electrical Reference2/LConn1 -- "l Km "/LConn2
  CB/RConn1 -- abc1/RConn1
  Electrical Reference4/LConn1 -- "l1 Km "/LConn2
  Electrical Reference3/LConn1 -- "l1 Km "/RConn2
  "l Km "/RConn1 -- "Fault "/LConn1 -- "l1 Km "/LConn1
  "l1 Km "/RConn1 -- CB/LConn1

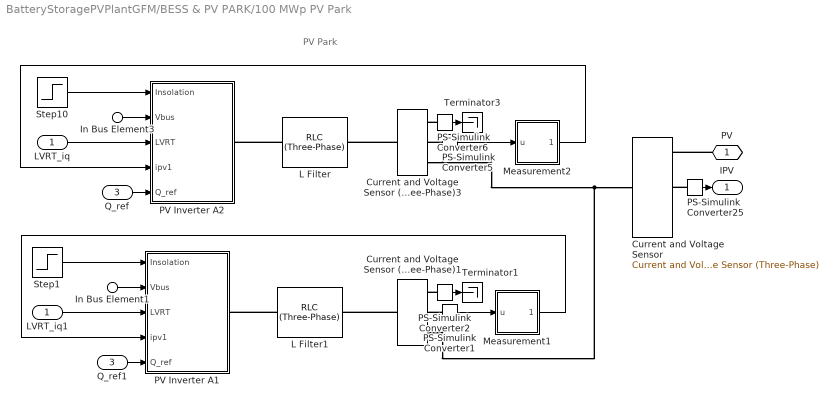
== system BatteryStoragePVPlantGFM/BESS & PV PARK/100 MWp PV Park ==
  note: PV Park
  LVRT_iq : Inport
  In Bus Element3 : Inport  Port=2  PortName=Vbus
  In Bus Element1 : Inport  Port=2  PortName=Vbus
  Q_ref : Inport  Port=3
  "Current and Voltage Sensor " : ee_lib/Sensors & Transducers/Current and Voltage Sensor (Three-Phase)  vMeasurementType=ee.enum.vmeasurement.lg  outputUnit=ee.enum.unit.pu  SRated=Base.MVA_base_new A*V  VRated=Base.KV_base_new V  I_specify=off  I_priority=None  I=[0, 0, 0] A  I_nominal_specify=off  I_nominal_unit=A  I_nominal_value=1  V_specify=off  V_priority=None  V=[0, 0, 0] V  V_nominal_specify=off  V_nominal_unit=V  V_nominal_value=1
      settings: InternalSimscapePortConfiguration="{\"Bottom\":[],\"Left\":[{\"id\":\"N1\",\"label\":\"~1\",\"type\":\"foundation.electrical.three_phase\"}],\"Right\":[{\"id\":\"V_output\",\"label\":\"V\",\"type\":\"output\"},{\"id\":\"I_output\",\"label\":\"I\",\"type\":\"output\"},{\"id\":\"N2\",\"label\":\"~2\",\"type\":\"foundation.electrical.three_phase\"}],\"Top\":[]}"
  Current and Voltage Sensor (Three-Phase)1 : ee_lib/Sensors & Transducers/Current and Voltage Sensor (Three-Phase)  vMeasurementType=ee.enum.vmeasurement.lg  outputUnit=ee.enum.unit.pu  SRated=Base.MVA_base_new A*V  VRated=Base.KV_base_new V  I_specify=off  I_priority=None  I=[0, 0, 0] A  I_nominal_specify=off  I_nominal_unit=A  I_nominal_value=1  V_specify=off  V_priority=None  V=[0, 0, 0] V  V_nominal_specify=off  V_nominal_unit=V  V_nominal_value=1
      settings: InternalSimscapePortConfiguration="{\"Bottom\":[],\"Left\":[{\"id\":\"N1\",\"label\":\"~1\",\"type\":\"foundation.electrical.three_phase\"}],\"Right\":[{\"id\":\"V_output\",\"label\":\"V\",\"type\":\"output\"},{\"id\":\"I_output\",\"label\":\"I\",\"type\":\"output\"},{\"id\":\"N2\",\"label\":\"~2\",\"type\":\"foundation.electrical.three_phase\"}],\"Top\":[]}"
  Current and Voltage Sensor (Three-Phase)3 : ee_lib/Sensors & Transducers/Current and Voltage Sensor (Three-Phase)  vMeasurementType=ee.enum.vmeasurement.lg  outputUnit=ee.enum.unit.pu  SRated=Base.MVA_base_new A*V  VRated=Base.KV_base_new V  I_specify=off  I_priority=None  I=[0, 0, 0] A  I_nominal_specify=off  I_nominal_unit=A  I_nominal_value=1  V_specify=off  V_priority=None  V=[0, 0, 0] V  V_nominal_specify=off  V_nominal_unit=V  V_nominal_value=1
      settings: InternalSimscapePortConfiguration="{\"Bottom\":[],\"Left\":[{\"id\":\"N1\",\"label\":\"~1\",\"type\":\"foundation.electrical.three_phase\"}],\"Right\":[{\"id\":\"V_output\",\"label\":\"V\",\"type\":\"output\"},{\"id\":\"I_output\",\"label\":\"I\",\"type\":\"output\"},{\"id\":\"N2\",\"label\":\"~2\",\"type\":\"foundation.electrical.three_phase\"}],\"Top\":[]}"
  L Filter : ee_lib/Passive/RLC Assemblies/RLC (Three-Phase)  component_structure=ee.enum.rlc.structure.L  R=1e-3 Ohm  L=PVInverter.L H  C=1e-6 F  R_parasitic=0 Ohm  G_parasitic=0 1/Ohm  IL_specify=off  IL_priority=High  IL=[0, 0, 0] A  IL_nominal_specify=off  IL_nominal_unit=A  IL_nominal_value=1  VC_specify=off  VC_priority=High  VC=[0, 0, 0] V  VC_nominal_specify=off  VC_nominal_unit=V  VC_nominal_value=1
      settings: InternalSimscapePortConfiguration="{\"Bottom\":[],\"Left\":[{\"id\":\"N1\",\"label\":\"~1\",\"type\":\"foundation.electrical.three_phase\"}],\"Right\":[{\"id\":\"N2\",\"label\":\"~2\",\"type\":\"foundation.electrical.three_phase\"}],\"Top\":[]}"
  L Filter1 : ee_lib/Passive/RLC Assemblies/RLC (Three-Phase)  component_structure=ee.enum.rlc.structure.L  R=1e-3 Ohm  L=PVInverter.L H  C=1e-6 F  R_parasitic=0 Ohm  G_parasitic=0 1/Ohm  IL_specify=off  IL_priority=High  IL=[0, 0, 0] A  IL_nominal_specify=off  IL_nominal_unit=A  IL_nominal_value=1  VC_specify=off  VC_priority=High  VC=[0, 0, 0] V  VC_nominal_specify=off  VC_nominal_unit=V  VC_nominal_value=1
      settings: InternalSimscapePortConfiguration="{\"Bottom\":[],\"Left\":[{\"id\":\"N1\",\"label\":\"~1\",\"type\":\"foundation.electrical.three_phase\"}],\"Right\":[{\"id\":\"N2\",\"label\":\"~2\",\"type\":\"foundation.electrical.three_phase\"}],\"Top\":[]}"
  LVRT_iq1 : InportShadow
  Measurement1 : Subsystem
  Measurement2 : Subsystem
  PS-Simulink Converter{1..2,5..6,25} (5 alike) : nesl_utility/PS-Simulink Converter  PhysicalDomain=network_engine_domain  SubClassName=ps_output  LeftPortType=input  RightPortType=output  PseudoPeriodic=off  Frequencies=[]  VectorFormat=inherit  Unit=inherit  AffineConversion=off
  PV Inverter A1 : Subsystem
  PV Inverter A2 : Subsystem
  Q_ref1 : InportShadow  Port=3
  Step1 : Step  Time=Scenario.Solar_flactuation_time  Before=Array.insolation  After=Array.insolation*0.7  SampleTime=Ts
  Step10 : Step  Time=Scenario.Solar_flactuation_time  Before=Array.insolation  After=Array.insolation*0.7  SampleTime=Ts
  Terminator1 : Terminator
  Terminator3 : Terminator
  PV : PMIOPort  Side=Left
  IPV : Outport
  wires:
  PS-Simulink Converter5/1 -> Measurement2/1(u)
  PS-Simulink Converter6/1 -> Terminator3/1
  Measurement2/1(ipv1) -> PV Inverter A2/4(ipv1)
  Step10/1 -> PV Inverter A2/1(Insolation)
  In Bus Element3/1 -> PV Inverter A2/2(Vbus)
  LVRT_iq/1 -> PV Inverter A2/3(LVRT)
  PS-Simulink Converter25/1 -> IPV/1
  Q_ref/1 -> PV Inverter A2/5(Q_ref)
  PS-Simulink Converter1/1 -> Measurement1/1(u)
  Q_ref1/1 -> PV Inverter A1/5(Q_ref)
  Step1/1 -> PV Inverter A1/1(Insolation)
  LVRT_iq1/1 -> PV Inverter A1/3(LVRT)
  PS-Simulink Converter2/1 -> Terminator1/1
  Measurement1/1(ipv1) -> PV Inverter A1/4(ipv1)
  In Bus Element1/1 -> PV Inverter A1/2(Vbus)
  connections:
  PS-Simulink Converter6/LConn1 -- Current and Voltage Sensor (Three-Phase)3/RConn1
  L Filter/LConn1 -- PV Inverter A2/RConn1
  PS-Simulink Converter5/LConn1 -- Current and Voltage Sensor (Three-Phase)3/RConn2
  PV/RConn1 -- "Current and Voltage Sensor "/RConn3
  PS-Simulink Converter25/LConn1 -- "Current and Voltage Sensor "/RConn2
  Current and Voltage Sensor (Three-Phase)3/LConn1 -- L Filter/RConn1
  Current and Voltage Sensor (Three-Phase)3/RConn3 -- "Current and Voltage Sensor "/LConn1 -- Current and Voltage Sensor (Three-Phase)1/RConn3
  PS-Simulink Converter2/LConn1 -- Current and Voltage Sensor (Three-Phase)1/RConn1
  L Filter1/LConn1 -- PV Inverter A1/RConn1
  PS-Simulink Converter1/LConn1 -- Current and Voltage Sensor (Three-Phase)1/RConn2
  Current and Voltage Sensor (Three-Phase)1/LConn1 -- L Filter1/RConn1

== system BatteryStoragePVPlantGFM/BESS & PV PARK/60 MWhr Battery Energy Storage ==
  In Bus Element : Inport  PortName=Vbus
  Input : Inport  Port=2
  Variant Subsystem : Subsystem  Variant=on
  GFL1 : PMIOPort  Side=Right
  Out Bus Element : Outport  PortName=Bat
  wires:
  In Bus Element/1 -> Variant Subsystem/1(Vbus)
  Input/1 -> Variant Subsystem/2(LVRT)
  Variant Subsystem/1(Bat) -> Out Bus Element/1
  connections:
  GFL1/RConn1 -- Variant Subsystem/LConn1

== system BatteryStoragePVPlantGFM/BESS & PV PARK/CB-3 ==
  Input : Inport
  Circuit Breaker Step off3 : ee_lib/Switches & Breakers/Circuit Breaker (Three-Phase)  R_closed=0.001 Ohm  G_open=1e-9 1/Ohm  threshold=0.5 V  breaker_behavior=ee.enum.switches.breakerBehavior.zeroCrossingEnable
      settings: InternalSimscapePortConfiguration="{\"Bottom\":[],\"Left\":[{\"id\":\"vT\",\"label\":\"vT\",\"type\":\"input\"},{\"id\":\"N1\",\"label\":\"~1\",\"type\":\"foundation.electrical.three_phase\"}],\"Right\":[{\"id\":\"N2\",\"label\":\"~2\",\"type\":\"foundation.electrical.three_phase\"}],\"Top\":[]}"
  Simulink-PS Converter3 : nesl_utility/Simulink-PS Converter  PhysicalDomain=network_engine_domain  SubClassName=ps_input  LeftPortType=input  RightPortType=output  PseudoPeriodic=off  Frequencies=[]  NoiseDistribution=none  NoiseParameters=[]  Unit=1  AffineConversion=off  FilteringAndDerivatives=zero  SimscapeFilterOrder=1  InputFilterTimeConstant=0.001  UdotUserProvided=1
  Conn2 : PMIOPort  Side=Left
  Conn1 : PMIOPort  Port=2  Side=Right
  wires:
  Input/1 -> Simulink-PS Converter3/1
  connections:
  Circuit Breaker Step off3/LConn2 -- Conn2/RConn1
  Circuit Breaker Step off3/LConn1 -- Simulink-PS Converter3/RConn1
  Circuit Breaker Step off3/RConn1 -- Conn1/RConn1

== system BatteryStoragePVPlantGFM/BESS & PV PARK/CB-4 ==
  Input : Inport
  Circuit Breaker Step off3 : ee_lib/Switches & Breakers/Circuit Breaker (Three-Phase)  R_closed=0.001 Ohm  G_open=1e-9 1/Ohm  threshold=0.5 V  breaker_behavior=ee.enum.switches.breakerBehavior.zeroCrossingEnable
      settings: InternalSimscapePortConfiguration="{\"Bottom\":[],\"Left\":[{\"id\":\"vT\",\"label\":\"vT\",\"type\":\"input\"},{\"id\":\"N1\",\"label\":\"~1\",\"type\":\"foundation.electrical.three_phase\"}],\"Right\":[{\"id\":\"N2\",\"label\":\"~2\",\"type\":\"foundation.electrical.three_phase\"}],\"Top\":[]}"
  Simulink-PS Converter3 : nesl_utility/Simulink-PS Converter  PhysicalDomain=network_engine_domain  SubClassName=ps_input  LeftPortType=input  RightPortType=output  PseudoPeriodic=off  Frequencies=[]  NoiseDistribution=none  NoiseParameters=[]  Unit=1  AffineConversion=off  FilteringAndDerivatives=zero  SimscapeFilterOrder=1  InputFilterTimeConstant=0.001  UdotUserProvided=1
  Conn2 : PMIOPort  Side=Left
  Conn1 : PMIOPort  Port=2  Side=Right
  wires:
  Input/1 -> Simulink-PS Converter3/1
  connections:
  Circuit Breaker Step off3/LConn2 -- Conn2/RConn1
  Circuit Breaker Step off3/LConn1 -- Simulink-PS Converter3/RConn1
  Circuit Breaker Step off3/RConn1 -- Conn1/RConn1

== system BatteryStoragePVPlantGFM/BESS & PV PARK/PV Plant Controller  ==
  In Bus Element14 : Inport  PortName=Vbus
  In Bus Element1 : Inport  PortName=Vbus
  In Bus Element3 : Inport  PortName=Vbus
  In Bus Element2 : Inport  Port=2  PortName=Bat
  In Bus Element4 : Inport  Port=2  PortName=Bat
  IPV : Inport  Port=3
  Bus Selector : BusSelector  OutputSignals=iq,breaker
  "Logging Signals " : Subsystem
  Power Measurements : Subsystem
  "Voltage VAR Control & LVRT, FRT" : Subsystem
      mask Display: image('$imagefile'); % Use "Edit Image" on toolstrip to change.
  LVRT_iq : Outport
  LVRT.breaker : Outport  Port=2
  signals : Outport  Port=3
  Q_ref : Outport  Port=4
  wires:
  In Bus Element14/1 -> "Voltage VAR Control & LVRT, FRT"/1(Vbus)
  In Bus Element1/1 -> Power Measurements/1(Vbus)
  In Bus Element2/1 -> Power Measurements/2(Bat)
  Power Measurements/1(Measure) -> "Logging Signals "/1(Measure)
  In Bus Element3/1 -> "Logging Signals "/2(Vbus)
  IPV/1 -> Power Measurements/3(ipv)
  In Bus Element4/1 -> "Logging Signals "/3(Bat)
  "Voltage VAR Control & LVRT, FRT"/1(LVRT) -> Bus Selector/1
  Bus Selector/1 -> LVRT_iq/1  "<iq>"
  Bus Selector/2 -> LVRT.breaker/1  "<breaker>"
  "Logging Signals "/1(Output) -> signals/1
  "Voltage VAR Control & LVRT, FRT"/2(Q_ref) -> Q_ref/1

== system BatteryStoragePVPlantGFM/Conventional Source/Measurements ==
  V : Inport
  I : Inport  Port=2
  Gain : Gain  Gain=1/Grid.MVA
  Gain1 : Gain  Gain=1/Grid.MVA
  Low-Pass Filter : eeGeneralControl/Low-Pass Filter (Discrete or Continuous)  K=1  T=PVController.t_sensor  B=inf  A=-inf  init_option=Inherited from block input  x0=0  Ts=Ts
  Low-Pass Filter1 : eeGeneralControl/Low-Pass Filter (Discrete or Continuous)  K=1  T=PVController.t_sensor  B=inf  A=-inf  init_option=Inherited from block input  x0=0  Ts=Ts
  Power Measurement (Three-Phase) : eePowerMeasurement/Power Measurement (Three-Phase)  LabelModeActiveChoice=Discrete  F=Grid.frequency  K=[1]  Seq=Positive  Ts=Ts
  Scope : Scope
  Unit Delay : UnitDelay  SampleTime=-1  HasFrameUpgradeWarning=on
  Unit Delay1 : UnitDelay  SampleTime=-1  HasFrameUpgradeWarning=on
  Out Bus Element : Outport  PortName=Grid  Element=Pe
  Out Bus Element1 : Outport  PortName=Grid  Element=Qe
  wires:
  Power Measurement (Three-Phase)/1 -> Scope/1, Gain/1
  I/1 -> Power Measurement (Three-Phase)/2
  Power Measurement (Three-Phase)/2 -> Gain1/1
  V/1 -> Power Measurement (Three-Phase)/1
  Gain/1 -> Low-Pass Filter/1
  Gain1/1 -> Low-Pass Filter1/1
  Low-Pass Filter/1 -> Unit Delay1/1
  Low-Pass Filter1/1 -> Unit Delay/1
  Unit Delay/1 -> Out Bus Element1/1
  Unit Delay1/1 -> Out Bus Element/1

== system BatteryStoragePVPlantGFM/Conventional Source/Variant Subsystem ==
  Grid : Inport
  Frequency Controlled Source : Subsystem  VariantControl=VSMFrequencyControlledSource
  Synchronous Machine : Subsystem  VariantControl=SynchronousMachine
  abc : PMIOPort  Side=Right
  Connection Port1 : PMIOPort  Port=2  Side=Left

== system BatteryStoragePVPlantGFM/MV Feeder (R//X=1.4) /CB1 ==
  Circuit Breaker Step off3 : ee_lib/Switches & Breakers/Circuit Breaker (Three-Phase)  R_closed=0.001 Ohm  G_open=1e-4 1/Ohm  threshold=0.5 V  breaker_behavior=ee.enum.switches.breakerBehavior.zeroCrossingEnable
      settings: InternalSimscapePortConfiguration="{\"Bottom\":[],\"Left\":[{\"id\":\"vT\",\"label\":\"vT\",\"type\":\"input\"},{\"id\":\"N1\",\"label\":\"~1\",\"type\":\"foundation.electrical.three_phase\"}],\"Right\":[{\"id\":\"N2\",\"label\":\"~2\",\"type\":\"foundation.electrical.three_phase\"}],\"Top\":[]}"
  Simulink-PS Converter3 : nesl_utility/Simulink-PS Converter  PhysicalDomain=network_engine_domain  SubClassName=ps_input  LeftPortType=input  RightPortType=output  PseudoPeriodic=off  Frequencies=[]  NoiseDistribution=none  NoiseParameters=[]  Unit=1  AffineConversion=off  FilteringAndDerivatives=zero  SimscapeFilterOrder=1  InputFilterTimeConstant=0.001  UdotUserProvided=1
  Step off3 : Step  Time=Scenario.Load_switching_time  Before=Load2CB_initial  After=Load2CB_final  SampleTime=Ts
  Conn1 : PMIOPort  Side=Right
  Conn2 : PMIOPort  Port=2  Side=Left
  wires:
  Step off3/1 -> Simulink-PS Converter3/1
  connections:
  Circuit Breaker Step off3/LConn2 -- Conn2/RConn1
  Circuit Breaker Step off3/LConn1 -- Simulink-PS Converter3/RConn1
  Circuit Breaker Step off3/RConn1 -- Conn1/RConn1

== system BatteryStoragePVPlantGFM/MV Feeder (R//X=1.4) /CB10 ==
  Circuit Breaker Step off3 : ee_lib/Switches & Breakers/Circuit Breaker (Three-Phase)  R_closed=0.001 Ohm  G_open=1e-4 1/Ohm  threshold=0.5 V  breaker_behavior=ee.enum.switches.breakerBehavior.zeroCrossingEnable
      settings: InternalSimscapePortConfiguration="{\"Bottom\":[],\"Left\":[{\"id\":\"vT\",\"label\":\"vT\",\"type\":\"input\"},{\"id\":\"N1\",\"label\":\"~1\",\"type\":\"foundation.electrical.three_phase\"}],\"Right\":[{\"id\":\"N2\",\"label\":\"~2\",\"type\":\"foundation.electrical.three_phase\"}],\"Top\":[]}"
  Simulink-PS Converter3 : nesl_utility/Simulink-PS Converter  PhysicalDomain=network_engine_domain  SubClassName=ps_input  LeftPortType=input  RightPortType=output  PseudoPeriodic=off  Frequencies=[]  NoiseDistribution=none  NoiseParameters=[]  Unit=1  AffineConversion=off  FilteringAndDerivatives=zero  SimscapeFilterOrder=1  InputFilterTimeConstant=0.001  UdotUserProvided=1
  Step off3 : Step  Time=0  After=0  SampleTime=Ts
  Conn1 : PMIOPort  Side=Right
  Conn2 : PMIOPort  Port=2  Side=Left
  wires:
  Step off3/1 -> Simulink-PS Converter3/1
  connections:
  Circuit Breaker Step off3/LConn2 -- Conn2/RConn1
  Circuit Breaker Step off3/LConn1 -- Simulink-PS Converter3/RConn1
  Circuit Breaker Step off3/RConn1 -- Conn1/RConn1

== system BatteryStoragePVPlantGFM/Measurements & PLL/PLL & Measurements ==
  V : Inport
  I : Inport  Port=2
  Measurement1 : Subsystem
  Measurement2 : Subsystem
  Subsystem : Subsystem
  Out Bus Element : Outport  PortName=Vbus  Element=Vq
  Out Bus Element1 : Outport  PortName=Vbus  Element=Vd
  Out Bus Element2 : Outport  PortName=Vbus  Element=w
  Out Bus Element3 : Outport  PortName=Vbus  Element=Theta
  Out Bus Element4 : Outport  PortName=Vbus  Element=Vmag
  Out Bus Element5 : Outport  PortName=Vbus  Element=Iq
  Out Bus Element6 : Outport  PortName=Vbus  Element=Id
  Out Bus Element7 : Outport  PortName=Vbus  Element=Iabc
  Out Bus Element8 : Outport  PortName=Vbus  Element=Vabc
  wires:
  V/1 -> Measurement2/1(u)
  Subsystem/2(freq) -> Out Bus Element2/1
  Subsystem/5(Vq) -> Out Bus Element/1
  Subsystem/3(angle) -> Out Bus Element3/1
  Subsystem/4(Vd) -> Out Bus Element1/1
  Measurement2/1(Vg) -> Out Bus Element8/1, Subsystem/1(Vabc)
  Subsystem/1(mag) -> Out Bus Element4/1
  I/1 -> Measurement1/1(u)
  Measurement1/1(Vg) -> Out Bus Element7/1, Subsystem/2(Iabc)
  Subsystem/7(Iq1) -> Out Bus Element5/1
  Subsystem/6(Id1) -> Out Bus Element6/1
